simulink model "pmsm_ctrl"  (R2025b)
settings: Solver=FixedStepDiscrete  StartTime=0.0  StopTime=1.2  FixedStep=5e-05  RelTol=1e-3

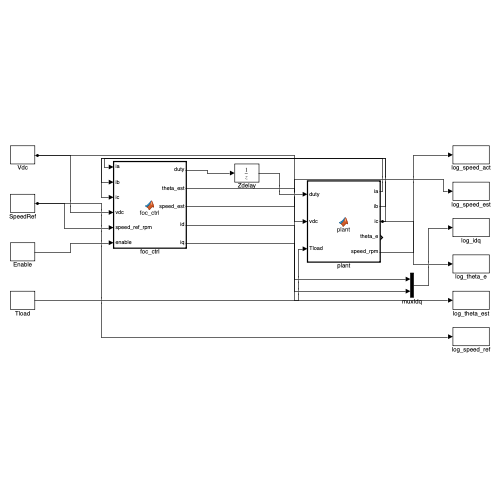
[thumbnail: Simulink's stored preview of the top-level diagram]
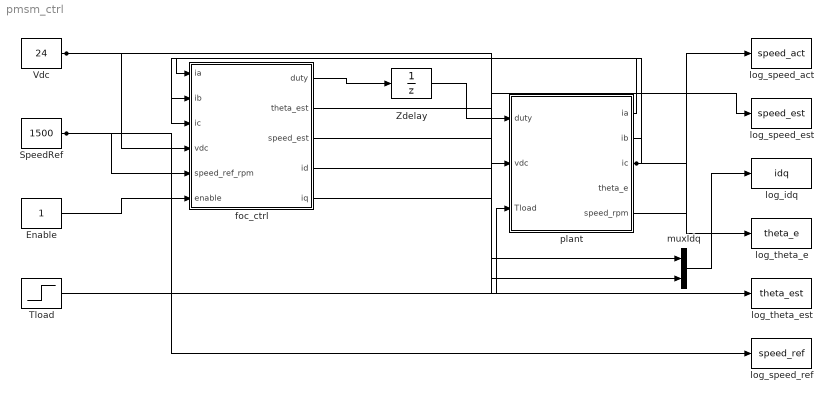
== system pmsm_ctrl ==
  Enable : Constant
  SpeedRef : Constant  Value=1500
  Tload : Step  Time=1.0  After=0.10  SampleTime=0
  Vdc : Constant  Value=24
  Zdelay : UnitDelay  InitialCondition=[0.5 0.5 0.5]  SampleTime=-1  HasFrameUpgradeWarning=on
  foc_ctrl : MATLAB Function  TreatAsAtomicUnit=on
  log_idq : ToWorkspace  VariableName=idq  SaveFormat=Timeseries  SampleTime=-1
  log_speed_act : ToWorkspace  VariableName=speed_act  SaveFormat=Timeseries  SampleTime=-1
  log_speed_est : ToWorkspace  VariableName=speed_est  SaveFormat=Timeseries  SampleTime=-1
  log_speed_ref : ToWorkspace  VariableName=speed_ref  SaveFormat=Timeseries  SampleTime=-1
  log_theta_e : ToWorkspace  VariableName=theta_e  SaveFormat=Timeseries  SampleTime=-1
  log_theta_est : ToWorkspace  VariableName=theta_est  SaveFormat=Timeseries  SampleTime=-1
  muxIdq : Mux  Inputs=2
  plant : MATLAB Function  TreatAsAtomicUnit=on
  wires:
  Vdc/1 -> foc_ctrl/4(vdc), plant/2(vdc)
  SpeedRef/1 -> foc_ctrl/5(speed_ref_rpm), log_speed_ref/1
  Enable/1 -> foc_ctrl/6(enable)
  foc_ctrl/1(duty) -> Zdelay/1
  Zdelay/1 -> plant/1(duty)
  Tload/1 -> plant/3(Tload)
  plant/1(ia) -> foc_ctrl/1(ia)
  plant/2(ib) -> foc_ctrl/2(ib)
  plant/3(ic) -> foc_ctrl/3(ic), log_theta_e/1
  plant/5(speed_rpm) -> log_speed_act/1
  foc_ctrl/3(speed_est) -> log_speed_est/1
  foc_ctrl/4(id) -> muxIdq/1
  foc_ctrl/5(iq) -> muxIdq/2
  muxIdq/1 -> log_idq/1
  foc_ctrl/2(theta_est) -> log_theta_est/1

== matlab function pmsm_ctrl/plant ==
function [ia, ib, ic, theta_e, speed_rpm] = plant(duty, vdc, Tload)
persistent st p initialized
if isempty(initialized)
    p = mc_params();
    st = pmsm_plant_init(p);
    initialized = true;
end
[ia, ib, ic, theta_e, speed_rpm, st] = pmsm_plant_step(duty, vdc, Tload, st, p);
end

== matlab function pmsm_ctrl/foc_ctrl ==
function [duty, theta_est, speed_est, id, iq] = foc_ctrl(ia, ib, ic, vdc, speed_ref_rpm, enable)
%#codegen
persistent st p initialized
if isempty(initialized)
    p = mc_params();
    st = foc_state_init(p);
    initialized = true;
end
[duty_s, dbg, st] = foc_controller_step(single(ia), single(ib), single(ic), single(vdc), single(speed_ref_rpm), single(enable), st, p);
% cast to double at the Simulink boundary (core stays single for STM32 C)
duty = double(duty_s);
theta_est = double(dbg(1));
speed_est = double(dbg(2));
id = double(dbg(3));
iq = double(dbg(4));
end
